simulink model "yh_play"  (Simulink 8.9)
settings: Solver=FixedStepAuto  StartTime=0.0  StopTime=Tf  FixedStep=delta_r  RelTol=1e-3  EnableMultiTasking=on
values from neighbouring files (symbols this model uses):
  A = [0    1             0       0 ... (first row only)    [Linear_system_main.m]
  A1 = [0    1             0       0 ... (first row only)    [Linear_system_main.m]
  B = [0 ... (first row only)    [Linear_system_main.m]
  B1 = [0 ... (first row only)    [Linear_system_main.m]
  C = [1 0 0 0]    [Linear_system_main.m]
  C1 = [1 0 0 0]    [Linear_system_main.m]
  decrease_threshold = increase_threshold/c    (= 3)    [Linear_system_main.m]
  delay_a = 0    [Linear_system_main.m]
  delay_KF = 0    [Linear_system_main.m]
  delay_MPC = 0    [Linear_system_main.m]
  delay_s = 0    [Linear_system_main.m]
  delta_r = 0.01    [Linear_system_main.m]
  delta_t = 0.2    [Linear_system_main.m]
  increase_threshold = 30    [Linear_system_main.m]
  test_period = 50    [Linear_system_main.m]
  TraceA = ones(1000000,1)    [Linear_system_main.m]
  uini = kini*Xini    [Linear_system_main.m]
  Xini = [0 3 2 0]'    [Linear_system_main.m]
  Xsp = [0,0,0,0]'    [Linear_system_main.m]
libraries: sldrtlib x1
settings Model: Creator=Rhine  LastModifiedBy=Yehan
settings OptimizationCC: ExpressionDepthLimit=2147483647
settings DebuggingCC: SolverPrmCheckMsg=warning

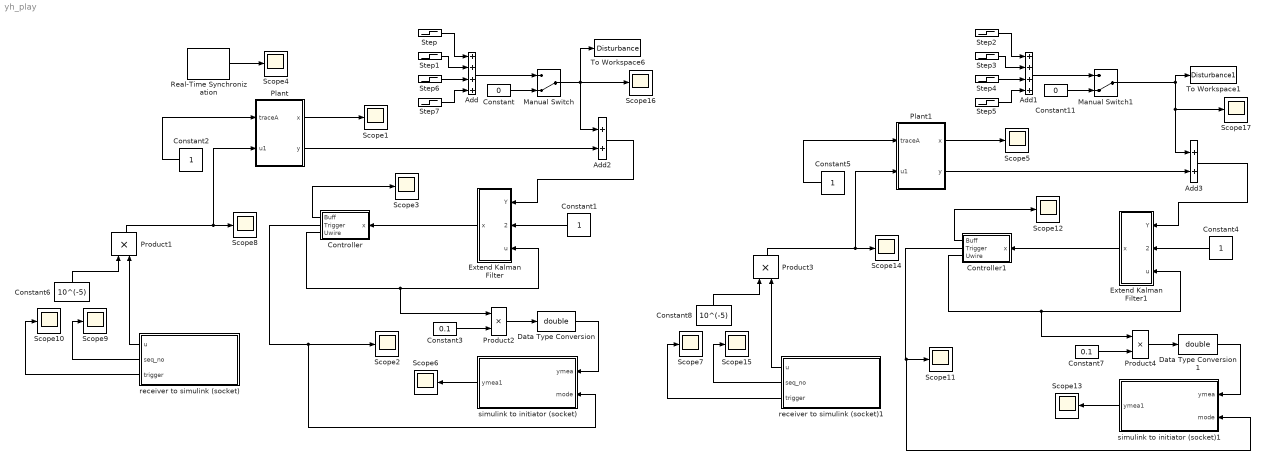
== system yh_play ==
  Add : Sum  Inputs=++++
  Add1 : Sum  Inputs=++++
  Add2 : Sum
  Add3 : Sum
  Constant : Constant  Value=0
  Constant{1..2,4..5} (4 alike) : Constant
  Constant11 : Constant  Value=0
  Constant3 : Constant  Value=0.1
  Constant6 : Constant  Value=10^(-5)
  Constant7 : Constant  Value=0.1
  Constant8 : Constant  Value=10^(-5)
  Controller : Subsystem
  Controller1 : Subsystem
  Data Type Conversion : DataTypeConversion  OutDataTypeStr=double
  Data Type Conversion1 : DataTypeConversion  OutDataTypeStr=double
  Extend Kalman Filter : Subsystem
  Extend Kalman Filter1 : Subsystem
  Manual Switch : ManualSwitch  CurrentSetting=0
  Manual Switch1 : ManualSwitch  CurrentSetting=0
  Plant : Subsystem
  Plant1 : Subsystem
  Product{1..4} (4 alike) : Product
  Real-Time Synchronization : sldrtlib/Real-Time Synchronization  SampleTime=delta_r  MaxMissedTicks=100000  ShowMissedTicks=on  YieldWhenWaiting=off
  Scope{1..17} (17 alike) : Scope
  Step : Step  Time=120  After=1.5  SampleTime=0
  Step1 : Step  Time=140  After=-1.5  SampleTime=0
  Step2 : Step  Time=120  After=3  SampleTime=0
  Step3 : Step  Time=140  After=-3  SampleTime=0
  Step4 : Step  Time=750  After=0  SampleTime=0
  Step5 : Step  Time=760  After=0  SampleTime=0
  Step6 : Step  Time=750  After=0  SampleTime=0
  Step7 : Step  Time=760  After=0  SampleTime=0
  To Workspace1 : ToWorkspace  VariableName=Disturbance1  SampleTime=-1
  To Workspace6 : ToWorkspace  VariableName=Disturbance  SampleTime=-1
  receiver to simulink (socket) : MATLAB Function  TreatAsAtomicUnit=on
  receiver to simulink (socket)1 : MATLAB Function  TreatAsAtomicUnit=on
  simulink to initiator (socket) : MATLAB Function  TreatAsAtomicUnit=on
  simulink to initiator (socket)1 : MATLAB Function  TreatAsAtomicUnit=on
  wires:
  Plant/1(x) -> Scope1/1
  Controller/3(Uwire) -> Product2/1, Extend Kalman Filter/3(u)
  Constant1/1 -> Extend Kalman Filter/2("trace 3 ")
  Constant2/1 -> Plant/1(traceA)
  Extend Kalman Filter/1(x) -> Controller/1(x)
  Real-Time Synchronization/1 -> Scope4/1
  simulink to initiator (socket)/1(ymea1) -> Scope6/1
  Data Type Conversion/1 -> simulink to initiator (socket)/1(ymea)
  Constant3/1 -> Product2/2
  Product2/1 -> Data Type Conversion/1
  Constant6/1 -> Product1/1
  Product1/1 -> Plant/2(u1), Scope8/1
  Controller/1(Buff) -> Scope3/1
  receiver to simulink (socket)/2(seq_no) -> Scope9/1
  receiver to simulink (socket)/3(trigger) -> Scope10/1
  receiver to simulink (socket)/1(u) -> Product1/2
  Controller1/2("Trigger ") -> simulink to initiator (socket)1/2(mode), Scope11/1
  Constant8/1 -> Product3/1
  receiver to simulink (socket)1/3(trigger) -> Scope7/1
  receiver to simulink (socket)1/2(seq_no) -> Scope15/1
  Controller1/1(Buff) -> Scope12/1
  Product4/1 -> Data Type Conversion1/1
  Product3/1 -> Plant1/2(u1), Scope14/1
  Plant1/1(x) -> Scope5/1
  Constant4/1 -> Extend Kalman Filter1/2("trace 3 ")
  Data Type Conversion1/1 -> simulink to initiator (socket)1/1(ymea)
  Constant7/1 -> Product4/2
  Constant5/1 -> Plant1/1(traceA)
  receiver to simulink (socket)1/1(u) -> Product3/2
  simulink to initiator (socket)1/1(ymea1) -> Scope13/1
  Extend Kalman Filter1/1(x) -> Controller1/1(x)
  Controller/2("Trigger ") -> simulink to initiator (socket)/2(mode), Scope2/1
  Controller1/3(Uwire) -> Product4/1, Extend Kalman Filter1/3(u)
  Step7/1 -> Add/4
  Manual Switch/1 -> Scope16/1, To Workspace6/1, Add2/1
  Add2/1 -> Extend Kalman Filter/1(Y)
  Plant/2(y) -> Add2/2
  Step/1 -> Add/1
  Step6/1 -> Add/3
  Constant/1 -> Manual Switch/2
  Add/1 -> Manual Switch/1
  Step1/1 -> Add/2
  Add3/1 -> Extend Kalman Filter1/1(Y)
  Plant1/2(y) -> Add3/2
  Step4/1 -> Add1/3
  Step3/1 -> Add1/2
  Step2/1 -> Add1/1
  Step5/1 -> Add1/4
  Constant11/1 -> Manual Switch1/2
  Add1/1 -> Manual Switch1/1
  Manual Switch1/1 -> Scope17/1, Add3/1, To Workspace1/1

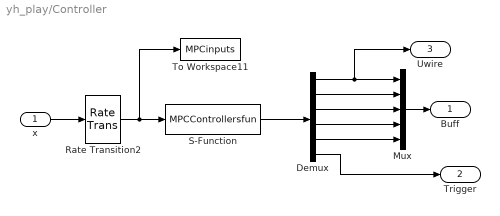
== system yh_play/Controller ==
  x : Inport
  Demux : Demux  Outputs=6
  Mux : Mux  Inputs=5
  Rate Transition2 : RateTransition  OutPortSampleTime=delta_r
  S-Function : S-Function  FunctionName=MPCControllersfun  Parameters=A,B,C,uini,Xsp,delta_t,delta_r,TraceA,increase_threshold,decrease_threshold,test_period,delay_s,delay_KF  SFunctionDeploymentMode=off  EnableBusSupport=off
  To Workspace11 : ToWorkspace  VariableName=MPCinputs  SampleTime=-1
  Buff : Outport
  "Trigger " : Outport  Port=2
  Uwire : Outport  Port=3
  wires:
  x/1 -> Rate Transition2/1
  S-Function/1 -> Demux/1
  Demux/1 -> Uwire/1, Mux/1
  Mux/1 -> Buff/1
  Demux/2 -> Mux/2
  Demux/3 -> Mux/3
  Demux/4 -> Mux/4
  Demux/5 -> Mux/5
  Rate Transition2/1 -> To Workspace11/1, S-Function/1
  Demux/6 -> "Trigger "/1

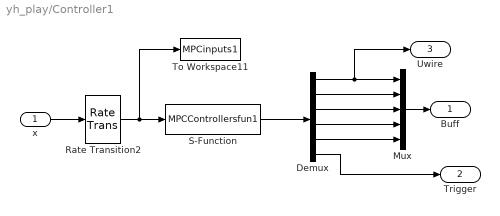
== system yh_play/Controller1 ==
  x : Inport
  Demux : Demux  Outputs=6
  Mux : Mux  Inputs=5
  Rate Transition2 : RateTransition  OutPortSampleTime=delta_r
  S-Function : S-Function  FunctionName=MPCControllersfun1  Parameters=A1,B1,C1,uini,Xsp,delta_t,delta_r,TraceA,increase_threshold,decrease_threshold,test_period,delay_s,delay_KF  SFunctionDeploymentMode=off  EnableBusSupport=off
  To Workspace11 : ToWorkspace  VariableName=MPCinputs1  SampleTime=-1
  Buff : Outport
  "Trigger " : Outport  Port=2
  Uwire : Outport  Port=3
  wires:
  x/1 -> Rate Transition2/1
  S-Function/1 -> Demux/1
  Demux/1 -> Uwire/1, Mux/1
  Mux/1 -> Buff/1
  Demux/2 -> Mux/2
  Demux/3 -> Mux/3
  Demux/4 -> Mux/4
  Demux/5 -> Mux/5
  Rate Transition2/1 -> To Workspace11/1, S-Function/1
  Demux/6 -> "Trigger "/1

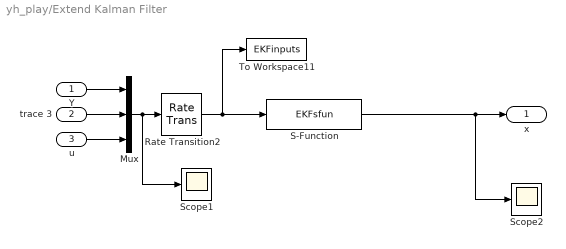
== system yh_play/Extend Kalman Filter ==
  Y : Inport
  "trace 3 " : Inport  Port=2
  u : Inport  Port=3
  Mux : Mux  Inputs=3
  Rate Transition2 : RateTransition  OutPortSampleTime=delta_r
  S-Function : S-Function  FunctionName=EKFsfun  Parameters=A,B,C,delta_t,delta_r,delay_s  SFunctionDeploymentMode=off  EnableBusSupport=off
  Scope1 : Scope
  Scope2 : Scope
  To Workspace11 : ToWorkspace  VariableName=EKFinputs  SampleTime=-1
  x : Outport
  wires:
  Y/1 -> Mux/1
  Mux/1 -> Scope1/1, Rate Transition2/1
  u/1 -> Mux/3
  S-Function/1 -> Scope2/1, x/1
  "trace 3 "/1 -> Mux/2
  Rate Transition2/1 -> To Workspace11/1, S-Function/1

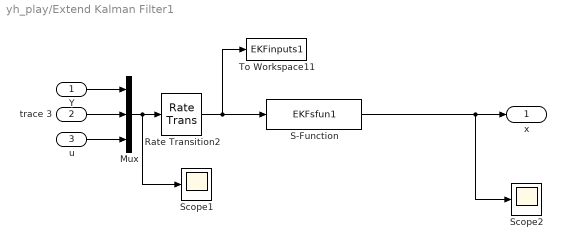
== system yh_play/Extend Kalman Filter1 ==
  Y : Inport
  "trace 3 " : Inport  Port=2
  u : Inport  Port=3
  Mux : Mux  Inputs=3
  Rate Transition2 : RateTransition  OutPortSampleTime=delta_r
  S-Function : S-Function  FunctionName=EKFsfun1  Parameters=A1,B1,C1,delta_t,delta_r,delay_s  SFunctionDeploymentMode=off  EnableBusSupport=off
  Scope1 : Scope
  Scope2 : Scope
  To Workspace11 : ToWorkspace  VariableName=EKFinputs1  SampleTime=-1
  x : Outport
  wires:
  Y/1 -> Mux/1
  Mux/1 -> Scope1/1, Rate Transition2/1
  u/1 -> Mux/3
  S-Function/1 -> Scope2/1, x/1
  "trace 3 "/1 -> Mux/2
  Rate Transition2/1 -> To Workspace11/1, S-Function/1

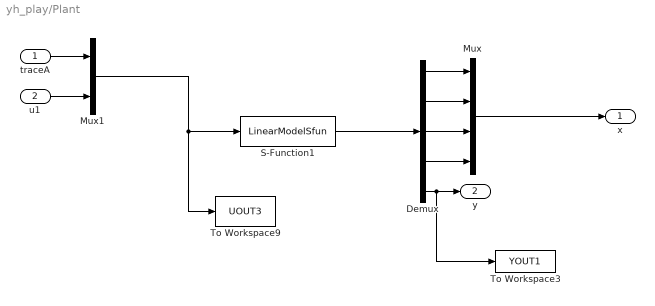
== system yh_play/Plant ==
  traceA : Inport
  u1 : Inport  Port=2
  Demux : Demux  Outputs=5
  Mux : Mux
  Mux1 : Mux  Inputs=2
  S-Function1 : S-Function  FunctionName=LinearModelSfun  Parameters=A,B,C,Xini,delta_t,delta_r,delay_s,delay_a,delay_KF,delay_MPC  SFunctionDeploymentMode=off  EnableBusSupport=off
  To Workspace3 : ToWorkspace  VariableName=YOUT1  SampleTime=-1
  To Workspace9 : ToWorkspace  VariableName=UOUT3  SampleTime=-1
  x : Outport
  y : Outport  Port=2
  wires:
  S-Function1/1 -> Demux/1
  Demux/1 -> Mux/1
  Demux/2 -> Mux/2
  Mux1/1 -> To Workspace9/1, S-Function1/1
  Demux/5 -> To Workspace3/1, y/1
  Demux/3 -> Mux/3
  Demux/4 -> Mux/4
  Mux/1 -> x/1
  u1/1 -> Mux1/2
  traceA/1 -> Mux1/1

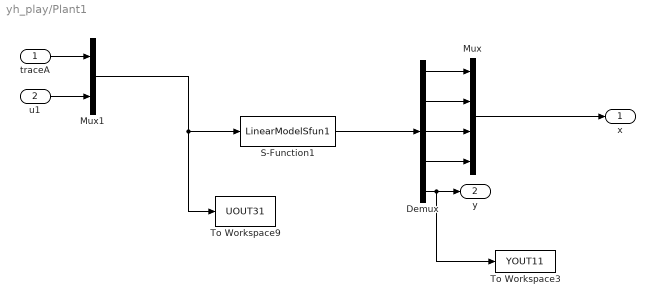
== system yh_play/Plant1 ==
  traceA : Inport
  u1 : Inport  Port=2
  Demux : Demux  Outputs=5
  Mux : Mux
  Mux1 : Mux  Inputs=2
  S-Function1 : S-Function  FunctionName=LinearModelSfun1  Parameters=A1,B1,C1,Xini,delta_t,delta_r,delay_s,delay_a,delay_KF,delay_MPC  SFunctionDeploymentMode=off  EnableBusSupport=off
  To Workspace3 : ToWorkspace  VariableName=YOUT11  SampleTime=-1
  To Workspace9 : ToWorkspace  VariableName=UOUT31  SampleTime=-1
  x : Outport
  y : Outport  Port=2
  wires:
  S-Function1/1 -> Demux/1
  Demux/1 -> Mux/1
  Demux/2 -> Mux/2
  Mux1/1 -> To Workspace9/1, S-Function1/1
  Demux/5 -> To Workspace3/1, y/1
  Demux/3 -> Mux/3
  Demux/4 -> Mux/4
  Mux/1 -> x/1
  u1/1 -> Mux1/2
  traceA/1 -> Mux1/1

== matlab function simulink to initiator (socket) ==
  data: ymea1 output double; ymea input double; mode input double
function ymea1   = Socket_block(ymea,mode)
% Inputs:
% ymea: measurement from structure
% Outputs:
% ymea1: measurement output
% ydelay: delay traces
% persistent i  % count

% allow these matlab functions to be used in Embedded Matlab block
%eml.extrinsic('python');
% eml.extrinsic('num2str');
% eml.extrinsic('str2num');
% eml.extrinsic('delay_summary');
% eml.extrinsic('disp');
eml.extrinsic('ps_aggregation');
% eml.extrinsic('for');
% eml.extrinsic('end');

% if isempty(i)
%     i = 0;
% end

results = ps_aggregation(ymea,mode);%here call TOSSIM Client ----yh

ymea1 = ymea;

== matlab function receiver to simulink (socket) ==
  data: u output double; seq_no output double; trigger output double
function [u,seq_no,trigger]   = Socket_block()
u=0;
trigger=0;
seq_no=0;
eml.extrinsic('ps_aggregation2');
% 
[u,trigger,seq_no] = ps_aggregation2();

% u1 = int32(results(1));
% seq_no1 = int32(results(2));
% trigger1 = int32(results(3));
% 
% % u=int32(u1);
% % seq_no=int32(seq_no1);
% % trigger=int32(trigger1);
% if results(1)>=-100000000
%     u1
% end
% u=0;
% seq_no=0;
% trigger=0;

== matlab function receiver to simulink (socket)1 ==
  data: u output double; seq_no output double; trigger output double
function [u,seq_no,trigger]   = Socket_block1()
u=0;
trigger=0;
seq_no=0;
eml.extrinsic('ps_aggregation21');
% 
[u,trigger,seq_no] = ps_aggregation21();

% u1 = int32(results(1));
% seq_no1 = int32(results(2));
% trigger1 = int32(results(3));
% 
% % u=int32(u1);
% % seq_no=int32(seq_no1);
% % trigger=int32(trigger1);
% if results(1)>=-100000000
%     u1
% end
% u=0;
% seq_no=0;
% trigger=0;

== matlab function simulink to initiator (socket)1 ==
  data: ymea1 output double; ymea input double; mode input double
function ymea1   = Socket_block1(ymea,mode)
% Inputs:
% ymea: measurement from structure
% Outputs:
% ymea1: measurement output
% ydelay: delay traces
% persistent i  % count

% allow these matlab functions to be used in Embedded Matlab block
%eml.extrinsic('python');
% eml.extrinsic('num2str');
% eml.extrinsic('str2num');
% eml.extrinsic('delay_summary');
% eml.extrinsic('disp');
eml.extrinsic('ps_aggregation1');
% eml.extrinsic('for');
% eml.extrinsic('end');

% if isempty(i)
%     i = 0;
% end

results = ps_aggregation1(ymea,mode);%here call TOSSIM Client ----yh

ymea1 = ymea;
